simulink model "SIL_position_controller"  (R2023b)
settings: Solver=FixedStepAuto  StartTime=0.0  StopTime=5  FixedStep=0.001  RelTol=1e-5  EnableMultiTasking=on
undefined symbols (not defined in the file): Ts
settings Model: SILPILSystemUnderTest=refmodels  ExtModeTrigDuration=10  Creator=paoli  LastModifiedBy=paoli
settings OptimizationCC: EnhancedBackFolding=on  PassReuseOutputArgsAs=Individual arguments  ZeroExternalMemoryAtStartup=off  ZeroInternalMemoryAtStartup=off  MaxStackSize=64  OptimizeBlockOrder=speed  DifferentSizesBufferReuse=on  OptimizationCustomize=off  EfficientTunableParamExpr=on
settings DebuggingCC: ParameterTunabilityLossMsg=error
settings HardwareCC: ProdBitPerPointer=32  ProdBitPerSizeT=32  ProdBitPerPtrDiffT=32  ProdLargestAtomicInteger=Long  ProdLargestAtomicFloat=Double  ProdWordSize=32  ProdLongLongMode=on  ProdHWDeviceType=ARM Compatible->ARM Cortex
settings SFSimCC: MATLABDynamicMemAlloc=off
settings RTWCC: Description=Embedded Coder  SystemTargetFile=ert.tlc  HardwareBoard=STM32 Nucleo F401RE  TemplateMakefile=ert_default_tmf  Toolchain=GNU Tools for ARM Embedded Processors  PortableWordSizes=on  CodeExecutionProfiling=on  CodeProfilingInstrumentation=coarse
settings CodeAppCC: ForceParamTrailComments=on  IgnoreCustomStorageClasses=off  OperatorAnnotations=on  SimulinkDataObjDesc=on  SFDataObjDesc=on  InsertBlockDesc=on
settings ERTTargetCC: ExtModeTransport=3  ExtModeStaticAlloc=on  ExtModeStaticAllocSize=2000  ExtModeMexFile=ext_xcp  ExtModeIntrfLevel=Level2 - Open

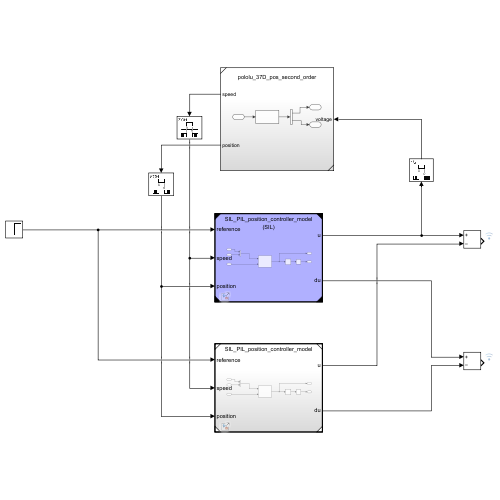
[thumbnail: Simulink's stored preview of the top-level diagram]
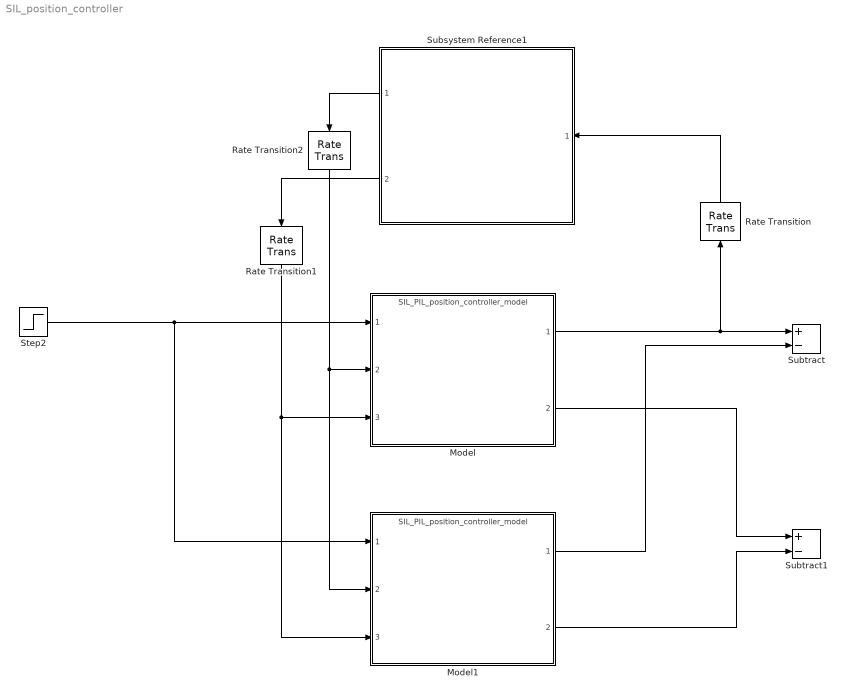
== system SIL_position_controller ==
  Model : ModelReference  ModelNameDialog=SIL_PIL_position_controller_model.slx  SimulationMode=Software-in-the-loop (SIL)  ModelReferenceVersion=1.4
  Model1 : ModelReference  ModelNameDialog=SIL_PIL_position_controller_model.slx  SimulationMode=Normal  ModelReferenceVersion=1.4
  Rate Transition : RateTransition
  Rate Transition1 : RateTransition
  Rate Transition2 : RateTransition
  Step2 : Step  Time=0  After=pi  SampleTime=Ts
  Subsystem Reference1 : Subsystem  ReferencedSubsystem=pololu_37D_pos_second_order
  Subtract : Sum  Inputs=+-
  Subtract1 : Sum  Inputs=+-
  wires:
  Model/1 -> Subtract/1, Rate Transition/1
  Subsystem Reference1/1 -> Rate Transition2/1
  Step2/1 -> Model1/1, Model/1
  Model1/1 -> Subtract/2
  Model/2 -> Subtract1/1
  Model1/2 -> Subtract1/2
  Rate Transition/1 -> Subsystem Reference1/1
  Rate Transition2/1 -> Model1/2, Model/2
  Subsystem Reference1/2 -> Rate Transition1/1
  Rate Transition1/1 -> Model1/3, Model/3
